simulink model "BANSHEE_SYSTEM"  (Simulink 8.1)
settings: Solver=ode1  StartTime=0.0  StopTime=inf  FixedStep=Ts  MaxStep=1e-3  RelTol=1e-3
PostLoadFcn:
  | Ts=100e-6; BANSHEE_init;
InitFcn:
  | Ts=100e-6; BANSHEE_init;
undefined symbols (not defined in the file or in its folder): cable_spec, F1, F2, F3, Feeder1_lib, Feeder2_lib, Feeder3_lib, Left, relay_housing_lib, SM_UtilityService, SS_F1_RELAY_HOUSING, SS_F2_RELAY_HOUSING, SS_F3_RELAY_HOUSING, SS_Feeder1, SS_Feeder2, SS_Feeder3, type, utility_service_lib, V
libraries: breaker_lib x50, relay_modbus_lib x42, rtio_generic_modbus x42, cables_lib x32, artemis x24, transformer_lib x24, Load_lib x18, ssn_lib x16, rtlab x11, powerlib_extras x3, powerlib x2, LoadProfiles_lib x1
(part 3 of 3)

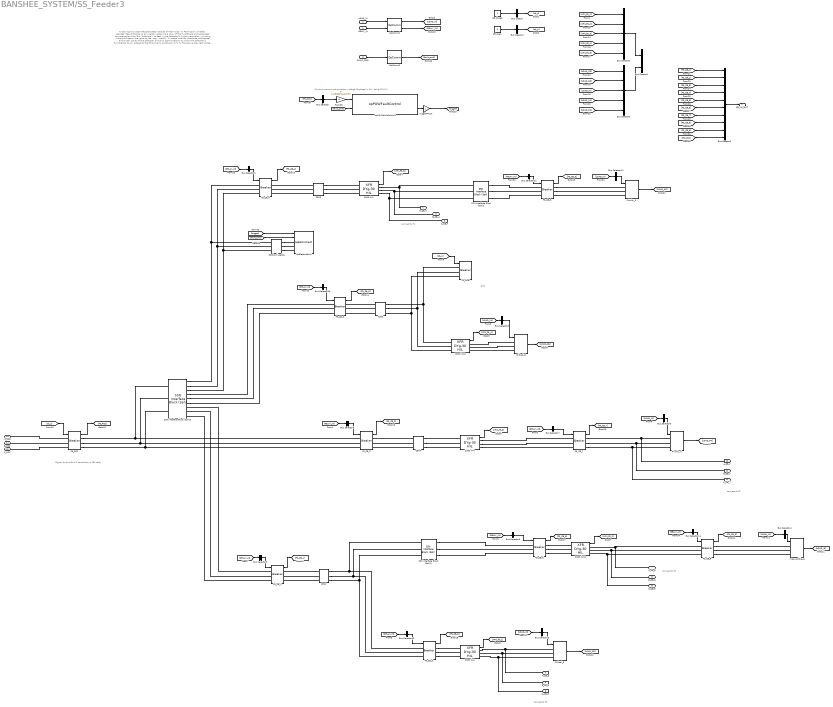
== system BANSHEE_SYSTEM/SS_Feeder3 ==
  note: Signal for this Cb will come from a SEL relay
  note: CHP
  note: connect to F2
  note: connect to F2
  note: connect to F2
  note: connect to F1
  note: % Copyright (c) 2016 Massachusetts Institute of Technology
      | % Permission is hereby granted, free of charge, to any person obtaining a copy of this
      | % software and associated documentation files (the "Software"), to deal in the Software
      | % without restriction, including without limitation the rights to use, copy, modify,
      | % merge, publish, distribute, sublicense, and/or sell copies of the Software, and to
      | % permit persons to whom the Software is furnished to do so, subject to the following
      | % conditions:
      | %
      | %
      | % The above copyright notice and this permission notice shall be included in
      | % all copies or substantial portions of the Software.
      | %
      | % THE SOFTWARE IS PROVIDED "AS IS", WITHOUT WARRANTY OF ANY KIND, EXPRESS OR IMPLIED,
      | % INCLUDING BUT NOT LIMITED TO THE WARRANTIES OF MERCHANTABILITY, FITNESS FOR A
      | % PARTICULAR PURPOSE AND NONINFRINGEMENT. IN NO EVENT SHALL THE AUTHORS OR COPYRIGHT
      | % HOLDERS BE LIABLE FOR ANY CLAIM, DAMAGES OR OTHER LIABILITY, WHETHER IN AN ACTION
      | % OF CONTRACT, TORT OR OTHERWISE, ARISING FROM, OUT OF OR IN CONNECTION WITH THE
      | % SOFTWARE OR THE USE OR OTHER DEALINGS IN THE SOFTWARE.
      | %
      | %
      | %%
  note: Point-on-wave synchronisation voltage (3-phase) in PU - Using 13.8 kV
  RELAY_IN : Inport
  LOAD_IN : Inport  Port=2
  FAULT_CMD : Inport  Port=3
  1000 kVA : transformer_lib/XFR DYg-30 HIL  Rating=1000  Vp=13800  Vs=480  Z=5.56  XR=5.49
  1000 kVA1 : transformer_lib/XFR DYg-30 HIL  Rating=1000  Vp=13800  Vs=480  Z=5.56  XR=5.49
  2000 kVA : transformer_lib/XFR DYg-30 HIL  Rating=2000  Vp=13800  Vs=480  Z=5.75  XR=5.7
  2000 kVA1 : transformer_lib/XFR DYg-30 HIL  Rating=2000  Vp=13800  Vs=480  Z=5.75  XR=5.7
  2500 kVA : transformer_lib/XFR DYg-30 HIL  Rating=2500  Vp=13800  Vs=480  Z=5.75  XR=6.6
  500kcmil_cable : cables_lib/500kcmil_cable  length=1  par_sets=1
  Bus Creator : BusCreator  Inputs=1
  Bus Creator1 : BusCreator  Inputs=1
  Bus Creator2 : BusCreator  Inputs=5
  Bus Creator3 : BusCreator  Inputs=5
  Bus Creator4 : BusCreator  Inputs=2
  Bus Creator5 : BusCreator  Inputs=10
  Bus Selector : BusSelector  OutputSignals=Vabc_bus
  Bus Selector1 : BusSelector  OutputSignals=F3_CB_4
  Bus Selector10 : BusSelector  OutputSignals=F3_CB_5
  Bus Selector11 : BusSelector  OutputSignals=P6
  Bus Selector12 : BusSelector  OutputSignals=F3_CB_9
  Bus Selector13 : BusSelector  OutputSignals=F3_CB_3
  Bus Selector14 : BusSelector  OutputSignals=F3_CB_8
  Bus Selector2 : BusSelector  OutputSignals=C6
  Bus Selector3 : BusSelector  OutputSignals=P4
  Bus Selector4 : BusSelector  OutputSignals=I6
  Bus Selector5 : BusSelector  OutputSignals=C5
  Bus Selector6 : BusSelector  OutputSignals=F3_CB_2
  Bus Selector7 : BusSelector  OutputSignals=F3_CB_7
  Bus Selector8 : BusSelector  OutputSignals=F3_CB_6
  Bus Selector9 : BusSelector  OutputSignals=F3_CB_1
  C301 : cables_lib/PI-Section  cable_spec=[cable_spec(13, :)]  line_length=2500  parallel_sets=1
  C302 : cables_lib/PI-Section  cable_spec=[cable_spec(11, :)]  line_length=2000  parallel_sets=1
  C303 : cables_lib/PI-Section  cable_spec=[cable_spec(13, :)]  line_length=2000  parallel_sets=1
  C304 : cables_lib/PI-Section  cable_spec=[cable_spec(11, :)]  line_length=1500  parallel_sets=2
  CB closed : Constant
  CB open : Constant  Value=0
  Critical_5 : Load_lib/Dynamic_Load  V=460  Ts=Ts
  Critical_6 : Load_lib/Dynamic_Load  V=460  Ts=Ts
  F3_CB_{1..9} (9 alike) : breaker_lib/Breaker  Ts=Ts
  F3_GCB : breaker_lib/Breaker  Ts=Ts
  F3_PCC : breaker_lib/Breaker  Ts=Ts
  Interruptible_6 : Load_lib/Dynamic_Load  V=460  Ts=Ts
  OpComm1 : rtlab/OpComm  nbport=2  groupe_acq=1  subsys_rate=0  st=0  Synchronization=on  Interpolation=on  Threshold=1.0  Missed_Data=off  Sim_Time=off  Samples=off  dynSigOut=off  from_console=0  warning_done=off  writeOpCommFile=off  Offset=off
  OpComm2 : rtlab/OpComm  nbport=1  groupe_acq=1  subsys_rate=0  st=0  Synchronization=on  Interpolation=on  Threshold=1.0  Missed_Data=off  Sim_Time=off  Samples=off  dynSigOut=off  from_console=1  warning_done=off  writeOpCommFile=off  Offset=off
  Priority_4 : Load_lib/Dynamic_Load  V=460  Ts=Ts
  Priority_6 : Load_lib/Dynamic_Load  V=460  Ts=Ts
  SSN Interface Block (3ph)1 : ssn_lib/SSN Interface Block (3ph)  nb_phase=3  nb_port=2  p1_type=V-type(Left)  p2_type=V-type (Right)  p3_type=V-type(Left)  p4_type=V-type(Left)  p5_type=V-type(Left)  p6_type=V-type(Left)  p7_type=V-type(Left)  p8_type=V-type(Left)  p9_type=V-type(Left)  p10_type=V-type(Left)  p11_type=V-type(Left)  p12_type=V-type(Left)  p13_type=V-type(Left)  p14_type=V-type(Left)  p15_type=V-type(Left)  p16_type=V-type(Left)  I_port_shunt_resistance=1e9
  SSN Interface Block (3ph)2 : ssn_lib/SSN Interface Block (3ph)  nb_phase=3  nb_port=2  p1_type=V-type(Left)  p2_type=V-type (Right)  p3_type=V-type(Left)  p4_type=V-type(Left)  p5_type=V-type(Left)  p6_type=V-type(Left)  p7_type=V-type(Left)  p8_type=V-type(Left)  p9_type=V-type(Left)  p10_type=V-type(Left)  p11_type=V-type(Left)  p12_type=V-type(Left)  p13_type=V-type(Left)  p14_type=V-type(Left)  p15_type=V-type(Left)  p16_type=V-type(Left)  I_port_shunt_resistance=1e9
  SSN Interface Block (3ph)5 : ssn_lib/SSN Interface Block (3ph)  nb_phase=3  nb_port=4  p1_type=V-type(Left)  p2_type=V-type (Right)  p3_type=V-type (Right)  p4_type=V-type (Right)  p5_type=V-type(Left)  p6_type=V-type(Left)  p7_type=V-type(Left)  p8_type=V-type(Left)  p9_type=V-type(Left)  p10_type=V-type(Left)  p11_type=V-type(Left)  p12_type=V-type(Left)  p13_type=V-type(Left)  p14_type=V-type(Left)  p15_type=V-type(Left)  p16_type=V-type(Left)  I_port_shunt_resistance=1e9
  a : Gain  Gain=1/(13800*sqrt(2/3))
  opElectricFault : artemis/Tools /POW faults/opElectricFault  FaultLocation=location 4  FaultResistance=0.0001  GroundResistance=0.0001  InitialStates=[0 0 0]  SnubberResistance=1e6  SnubberCapacitance=inf
  opPOWFaultControl1 : artemis/Tools /POW faults/opPOWFaultControl  Ts=Ts  usePLL=off  Fgrid=60  PLL_k=[180 3200 1]  vol_sel=1: rising zero-corssing  SyncPhase_menu=A  T_acq=0.8
  triggerFAULT : Gain
  A_CB_4 : PMIOPort  Port=1  Side=Right
  B_CB_4 : PMIOPort  Port=2  Side=Right
  C_CB_4 : PMIOPort  Port=3  Side=Right
  A_CB_5 : PMIOPort  Port=4  Side=Right
  B_CB_5 : PMIOPort  Port=5  Side=Right
  C_CB_5 : PMIOPort  Port=6  Side=Right
  A_CB_6 : PMIOPort  Port=7  Side=Right
  B_CB_6 : PMIOPort  Port=8  Side=Right
  C_CB_6 : PMIOPort  Port=9  Side=Right
  A_CB_7 : PMIOPort  Port=10  Side=Right
  B_CB_7 : PMIOPort  Port=11  Side=Right
  C_CB_7 : PMIOPort  Port=12  Side=Right
  A_PCC : PMIOPort  Port=13  Side=Left
  B_PCC : PMIOPort  Port=14  Side=Left
  C_PCC : PMIOPort  Port=15  Side=Left
  CB_MS_OUT : Outport
  wires:
  CB closed/1 -> Bus Creator/1  "Logic_trip"
  Bus Creator/1 -> [cb_c]
  Bus Creator1/1 -> [cb_o]
  Bus Selector1/1 -> F3_CB_4/1  "<F3_CB_4>"
  CB open/1 -> Bus Creator1/1  "Logic_trip"
  LOAD_IN/1 -> OpComm1/1
  OpComm1/1 -> [LOAD_IN]
  [LOAD_IN] -> Bus Selector2/1
  [LOAD_IN] -> Bus Selector3/1
  [LOAD_IN] -> Bus Selector4/1
  [LOAD_IN] -> Bus Selector5/1
  Bus Selector2/1 -> Critical_6/1  "<C6>"
  Bus Selector3/1 -> Priority_4/1  "<P4>"
  Bus Selector4/1 -> Interruptible_6/1  "<I6>"
  Bus Selector5/1 -> Critical_5/1  "<C5>"
  2000 kVA/1 -> [XFM_F3_1]
  2000 kVA1/1 -> [XFM_F3_2]
  1000 kVA/1 -> [XFM_F3_3]
  1000 kVA1/1 -> [XFM_F3_4]
  [XFM_F3_2] -> Bus Creator2/2  "F3_X2"
  [XFM_F3_1] -> Bus Creator2/1  "F3_X1"
  [XFM_F3_5] -> Bus Creator2/5  "F3_X5"
  [XFM_F3_3] -> Bus Creator2/3  "F3_X3"
  [XFM_F3_4] -> Bus Creator2/4  "F3_X4"
  Critical_6/1 -> [LOAD_C6]
  Priority_4/1 -> [LOAD_P4]
  Interruptible_6/1 -> [LOAD_I6]
  Critical_5/1 -> [LOAD_C5]
  [LOAD_C6] -> Bus Creator3/2  "F3_C6"
  [LOAD_C5] -> Bus Creator3/1  "F3_C5"
  [LOAD_I6] -> Bus Creator3/3  "F3_I6"
  [LOAD_P4] -> Bus Creator3/4  "F3_P4"
  Bus Creator2/1 -> Bus Creator4/1  "XFR"
  Bus Creator3/1 -> Bus Creator4/2  "LOAD"
  F3_CB_4/1 -> [F3_CB_4]
  F3_CB_3/1 -> [F3_CB_3]
  F3_CB_2/1 -> [F3_CB_2]
  F3_CB_6/1 -> [F3_CB_6]
  F3_CB_1/1 -> [F3_CB_1]
  F3_CB_5/1 -> [F3_CB_5]
  [F3_CB_1] -> Bus Creator5/1  "F3_CB_1"
  [F3_CB_5] -> Bus Creator5/5  "F3_CB_5"
  [F3_CB_7] -> Bus Creator5/7  "F3_CB_7"
  [F3_CB_6] -> Bus Creator5/6  "F3_CB_6"
  [F3_CB_3] -> Bus Creator5/3  "F3_CB_3"
  [F3_CB_2] -> Bus Creator5/2  "F3_CB_2"
  [F3_CB_4] -> Bus Creator5/4  "F3_CB_4"
  Bus Creator5/1 -> CB_MS_OUT/1
  [RELAY_IN] -> Bus Selector1/1
  RELAY_IN/1 -> OpComm1/2
  OpComm1/2 -> [RELAY_IN]
  Bus Selector6/1 -> F3_CB_2/1  "<F3_CB_2>"
  [RELAY_IN] -> Bus Selector6/1
  Bus Selector7/1 -> F3_CB_7/1  "<F3_CB_7>"
  [RELAY_IN] -> Bus Selector7/1
  Bus Selector8/1 -> F3_CB_6/1  "<F3_CB_6>"
  [RELAY_IN] -> Bus Selector8/1
  Bus Selector9/1 -> F3_CB_1/1  "<F3_CB_1>"
  [RELAY_IN] -> Bus Selector9/1
  Bus Selector10/1 -> F3_CB_5/1  "<F3_CB_5>"
  [RELAY_IN] -> Bus Selector10/1
  Bus Selector13/1 -> F3_CB_3/1  "<F3_CB_3>"
  [RELAY_IN] -> Bus Selector13/1
  [cb_c] -> F3_PCC/1
  [cb_o] -> F3_GCB/1
  2500 kVA/1 -> [XFM_F3_5]
  F3_CB_7/1 -> [F3_CB_7]
  F3_PCC/1 -> [F3_PCC]
  [F3_PCC] -> Bus Creator5/10  "F3_PCC"
  [LOAD_IN] -> Bus Selector11/1
  Bus Selector11/1 -> Priority_6/1  "<P6>"
  Priority_6/1 -> [LOAD_P6]
  [LOAD_P6] -> Bus Creator3/5  "F3_P6"
  F3_CB_9/1 -> [F3_CB_9]
  Bus Selector12/1 -> F3_CB_9/1  "<F3_CB_9>"
  [RELAY_IN] -> Bus Selector12/1
  F3_CB_8/1 -> [F3_CB_8]
  Bus Selector14/1 -> F3_CB_8/1  "<F3_CB_8>"
  [RELAY_IN] -> Bus Selector14/1
  [F3_CB_8] -> Bus Creator5/8  "F3_CB_8"
  [F3_CB_9] -> Bus Creator5/9  "F3_CB_9"
  [fault_cmd] -> opPOWFaultControl1/2
  opPOWFaultControl1/2 -> triggerFAULT/1
  triggerFAULT/1 -> [trigger]  "triggerFAULTsig"
  [F3_PCC] -> Bus Selector/1
  Bus Selector/1 -> a/1  "<Vabc_bus>"
  a/1 -> opPOWFaultControl1/1
  [fault_cmd] -> opElectricFault/2
  [trigger] -> opElectricFault/1
  OpComm2/1 -> [fault_cmd]
  FAULT_CMD/1 -> OpComm2/1
  connections:
  F3_CB_5/LConn1 -- C301/RConn1 -- SSN Interface Block (3ph)1/LConn1
  F3_CB_6/RConn3 -- 2000 kVA1/LConn3
  Critical_6/LConn2 -- 1000 kVA1/RConn2
  C301/LConn2 -- F3_CB_1/RConn2
  Critical_6/LConn1 -- 1000 kVA1/RConn1
  F3_CB_5/LConn3 -- C301/RConn3 -- SSN Interface Block (3ph)1/LConn3
  Critical_6/LConn3 -- 1000 kVA1/RConn3
  C301/LConn3 -- F3_CB_1/RConn3
  C304/LConn1 -- F3_CB_2/RConn1
  1000 kVA1/LConn3 -- C302/RConn3 -- F3_GCB/LConn3
  C302/LConn2 -- F3_CB_3/RConn2
  1000 kVA1/LConn1 -- C302/RConn1 -- F3_GCB/LConn1
  F3_CB_6/RConn2 -- 2000 kVA1/LConn2
  1000 kVA1/LConn2 -- C302/RConn2 -- F3_GCB/LConn2
  C301/LConn1 -- F3_CB_1/RConn1
  F3_CB_5/RConn2 -- 2000 kVA/LConn2
  C302/LConn3 -- F3_CB_3/RConn3
  F3_CB_5/LConn2 -- C301/RConn2 -- SSN Interface Block (3ph)1/LConn2
  C304/LConn2 -- F3_CB_2/RConn2
  F3_CB_6/RConn1 -- 2000 kVA1/LConn1
  C302/LConn1 -- F3_CB_3/RConn1
  F3_CB_5/RConn1 -- 2000 kVA/LConn1
  F3_CB_5/RConn3 -- 2000 kVA/LConn3
  C304/LConn3 -- F3_CB_2/RConn3
  F3_CB_7/RConn1 -- A_CB_7/RConn1 -- Priority_4/LConn1
  F3_CB_7/RConn3 -- C_CB_7/RConn1 -- Priority_4/LConn3
  F3_CB_7/RConn2 -- B_CB_7/RConn1 -- Priority_4/LConn2
  F3_CB_8/LConn1 -- A_CB_6/RConn1 -- 2000 kVA1/RConn1
  2000 kVA1/RConn3 -- C_CB_6/RConn1 -- F3_CB_8/LConn3
  F3_CB_8/LConn2 -- B_CB_6/RConn1 -- 2000 kVA1/RConn2
  Critical_5/LConn1 -- A_CB_5/RConn1 -- 2000 kVA/RConn1
  2000 kVA/RConn3 -- C_CB_5/RConn1 -- Critical_5/LConn3
  2000 kVA/RConn2 -- B_CB_5/RConn1 -- Critical_5/LConn2
  2500 kVA/RConn1 -- SSN Interface Block (3ph)2/LConn1 -- A_CB_4/RConn1
  2500 kVA/RConn3 -- SSN Interface Block (3ph)2/LConn3 -- C_CB_4/RConn1
  2500 kVA/RConn2 -- SSN Interface Block (3ph)2/LConn2 -- B_CB_4/RConn1
  C304/RConn2 -- 1000 kVA/LConn2
  C304/RConn3 -- 1000 kVA/LConn3
  C304/RConn1 -- 1000 kVA/LConn1
  1000 kVA/RConn3 -- F3_CB_7/LConn3
  1000 kVA/RConn2 -- F3_CB_7/LConn2
  1000 kVA/RConn1 -- F3_CB_7/LConn1
  F3_CB_9/RConn1 -- Priority_6/LConn1
  F3_CB_9/RConn2 -- Priority_6/LConn2
  F3_CB_9/RConn3 -- Priority_6/LConn3
  F3_CB_8/RConn1 -- Interruptible_6/LConn1
  F3_CB_8/RConn2 -- Interruptible_6/LConn2
  F3_CB_8/RConn3 -- Interruptible_6/LConn3
  SSN Interface Block (3ph)5/RConn1 -- 500kcmil_cable/LConn1 -- F3_CB_4/LConn1
  SSN Interface Block (3ph)5/RConn3 -- 500kcmil_cable/LConn3 -- F3_CB_4/LConn3
  SSN Interface Block (3ph)5/RConn2 -- 500kcmil_cable/LConn2 -- F3_CB_4/LConn2
  SSN Interface Block (3ph)5/RConn4 -- F3_CB_3/LConn1
  SSN Interface Block (3ph)5/RConn6 -- F3_CB_3/LConn3
  SSN Interface Block (3ph)5/RConn5 -- F3_CB_3/LConn2
  F3_CB_1/LConn1 -- SSN Interface Block (3ph)5/RConn7
  F3_CB_1/LConn2 -- SSN Interface Block (3ph)5/RConn8
  F3_CB_1/LConn3 -- SSN Interface Block (3ph)5/RConn9
  SSN Interface Block (3ph)1/RConn2 -- F3_CB_6/LConn2
  SSN Interface Block (3ph)1/RConn1 -- F3_CB_6/LConn1
  SSN Interface Block (3ph)1/RConn3 -- F3_CB_6/LConn3
  C303/LConn1 -- F3_CB_4/RConn1
  C303/LConn2 -- F3_CB_4/RConn2
  C303/LConn3 -- F3_CB_4/RConn3
  C303/RConn2 -- 2500 kVA/LConn2
  C303/RConn3 -- 2500 kVA/LConn3
  C303/RConn1 -- 2500 kVA/LConn1
  F3_PCC/LConn2 -- B_PCC/RConn1
  F3_PCC/LConn3 -- C_PCC/RConn1
  F3_PCC/LConn1 -- A_PCC/RConn1
  F3_PCC/RConn1 -- F3_CB_2/LConn1 -- SSN Interface Block (3ph)5/LConn1
  F3_PCC/RConn3 -- F3_CB_2/LConn3 -- SSN Interface Block (3ph)5/LConn3
  F3_PCC/RConn2 -- F3_CB_2/LConn2 -- SSN Interface Block (3ph)5/LConn2
  500kcmil_cable/RConn2 -- opElectricFault/LConn2
  500kcmil_cable/RConn3 -- opElectricFault/LConn3
  500kcmil_cable/RConn1 -- opElectricFault/LConn1
  SSN Interface Block (3ph)2/RConn2 -- F3_CB_9/LConn2
  SSN Interface Block (3ph)2/RConn3 -- F3_CB_9/LConn3
  SSN Interface Block (3ph)2/RConn1 -- F3_CB_9/LConn1

== system BANSHEE_SYSTEM/SC_ctrl/Overall ==
  F1 : Inport
  F2 : Inport  Port=2
  F3 : Inport  Port=3
  Iabc : Scope  NumInputPorts=3
      settings: ShowLegends=on  TimeRange=10  YMin=0~0~2  YMax=47.5~650~21  Decimation=10
  Vpu : Scope  NumInputPorts=3
      settings: ShowLegends=on  TimeRange=10  YMin=0~0~0  YMax=1.4~1.4~1.4  SaveName=ScopeData3  Decimation=10
  currents : Subsystem
  voltages : Subsystem
  wires:
  voltages/1(oF1) -> Vpu/1
  voltages/2(oF2) -> Vpu/2
  voltages/3(oF3) -> Vpu/3
  currents/1(oF1) -> Iabc/1
  currents/2(oF2) -> Iabc/2
  currents/3(oF3) -> Iabc/3
  F3/1 -> voltages/3(F3), currents/3(F3)
  F2/1 -> currents/2(F2), voltages/2(F2)
  F1/1 -> voltages/1(F1), currents/1(F1)

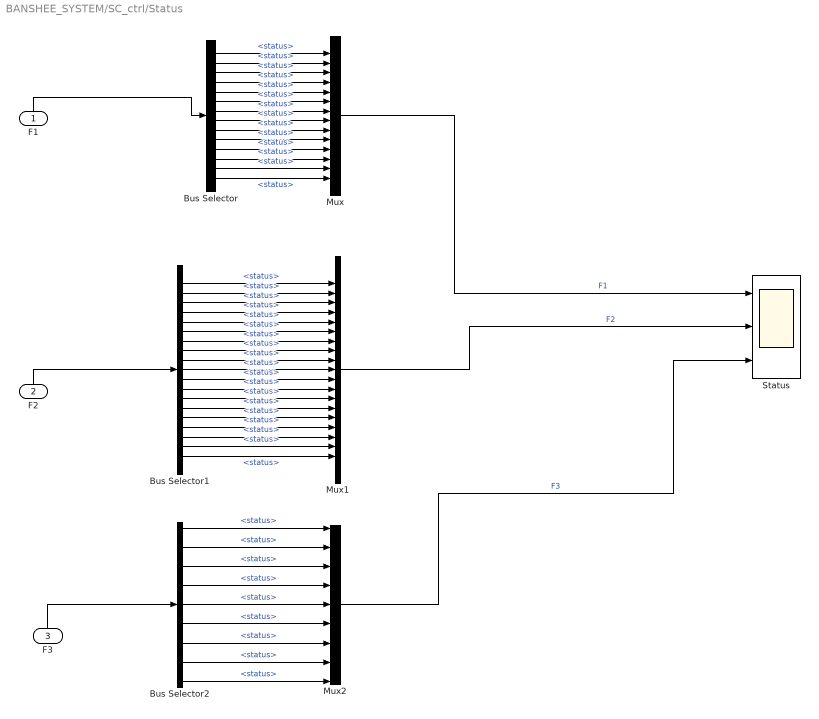
== system BANSHEE_SYSTEM/SC_ctrl/Status ==
  F1 : Inport
  F2 : Inport  Port=2
  F3 : Inport  Port=3
  Bus Selector : BusSelector  OutputSignals=F1_CB_1.m.status,F1_CB_2.m.status,F1_CB_3.m.status,F1_CB_4.m.status,F1_CB_5.m.status,F1_CB_6.m.status,F1_CB_7.m.status,F1_CB_8.m.status,F1_CB_9.m.status,F1_CB_10.m.status,F1_CB_11.m.status,F1_CB_12.m.status,F1_CB_13.m.status,F1_CB_14.m.status
  Bus Selector1 : BusSelector  OutputSignals=F2_CB_1.m.status,F2_CB_2.m.status,F2_CB_3.m.status,F2_CB_4.m.status,F2_CB_5.m.status,F2_CB_6.m.status,F2_CB_7.m.status,F2_CB_8.m.status,F2_CB_9.m.status,F2_CB_10.m.status,F2_CB_11.m.status,F2_CB_12.m.status,F2_CB_13.m.status,F2_CB_14.m.status,F2_CB_15.m.status,F2_CB_16.m.status,F2_CB_17.m.status,F2_CB_18.m.status,F2_CB_19.m.status
  Bus Selector2 : BusSelector  OutputSignals=F3_CB_1.m.status,F3_CB_2.m.status,F3_CB_3.m.status,F3_CB_4.m.status,F3_CB_5.m.status,F3_CB_6.m.status,F3_CB_7.m.status,F3_CB_8.m.status,F3_CB_9.m.status
  Mux : Mux  Inputs=14
  Mux1 : Mux  Inputs=19
  Mux2 : Mux  Inputs=9
  Status : Scope  NumInputPorts=3
      settings: ShowLegends=on  TimeRange=0.4  YMin=2~2~2.85  YMax=3~19~3.15  SaveName=ScopeData3  Decimation=20
  wires:
  Mux/1 -> Status/1  "F1"
  F1/1 -> Bus Selector/1
  Mux1/1 -> Status/2  "F2"
  F2/1 -> Bus Selector1/1
  Mux2/1 -> Status/3  "F3"
  F3/1 -> Bus Selector2/1
  Bus Selector1/3 -> Mux1/3  "<status>"
  Bus Selector1/13 -> Mux1/13  "<status>"
  Bus Selector1/8 -> Mux1/8  "<status>"
  Bus Selector1/4 -> Mux1/4  "<status>"
  Bus Selector1/6 -> Mux1/6  "<status>"
  Bus Selector1/2 -> Mux1/2  "<status>"
  Bus Selector1/7 -> Mux1/7  "<status>"
  Bus Selector1/10 -> Mux1/10  "<status>"
  Bus Selector1/12 -> Mux1/12  "<status>"
  Bus Selector1/1 -> Mux1/1  "<status>"
  Bus Selector1/5 -> Mux1/5  "<status>"
  Bus Selector1/14 -> Mux1/14  "<status>"
  Bus Selector1/9 -> Mux1/9  "<status>"
  Bus Selector1/11 -> Mux1/11  "<status>"
  Bus Selector1/17 -> Mux1/17  "<status>"
  Bus Selector1/16 -> Mux1/16  "<status>"
  Bus Selector1/15 -> Mux1/15  "<status>"
  Bus Selector1/18 -> Mux1/18  "<status>"
  Bus Selector1/19 -> Mux1/19  "<status>"
  Bus Selector/4 -> Mux/4  "<status>"
  Bus Selector/10 -> Mux/10  "<status>"
  Bus Selector/8 -> Mux/8  "<status>"
  Bus Selector/1 -> Mux/1  "<status>"
  Bus Selector/7 -> Mux/7  "<status>"
  Bus Selector/12 -> Mux/12  "<status>"
  Bus Selector/5 -> Mux/5  "<status>"
  Bus Selector/9 -> Mux/9  "<status>"
  Bus Selector/2 -> Mux/2  "<status>"
  Bus Selector/3 -> Mux/3  "<status>"
  Bus Selector/6 -> Mux/6  "<status>"
  Bus Selector/11 -> Mux/11  "<status>"
  Bus Selector/13 -> Mux/13  "<status>"
  Bus Selector/14 -> Mux/14  "<status>"
  Bus Selector2/6 -> Mux2/6  "<status>"
  Bus Selector2/5 -> Mux2/5  "<status>"
  Bus Selector2/7 -> Mux2/7  "<status>"
  Bus Selector2/4 -> Mux2/4  "<status>"
  Bus Selector2/8 -> Mux2/8  "<status>"
  Bus Selector2/3 -> Mux2/3  "<status>"
  Bus Selector2/9 -> Mux2/9  "<status>"
  Bus Selector2/2 -> Mux2/2  "<status>"
  Bus Selector2/1 -> Mux2/1  "<status>"

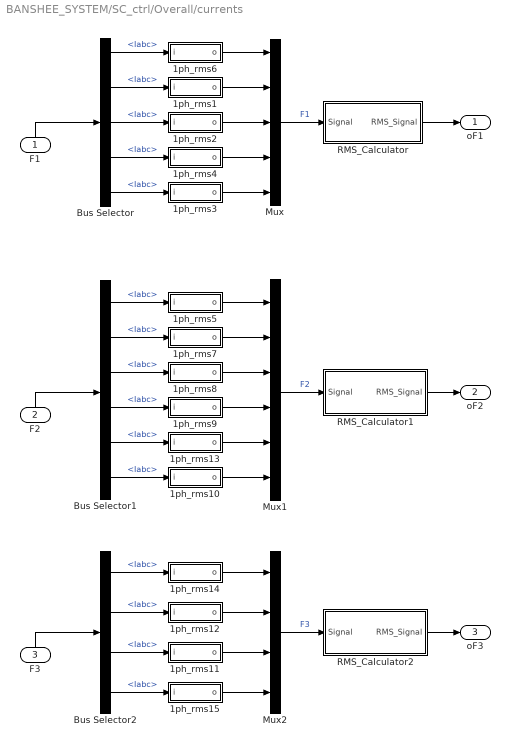
== system BANSHEE_SYSTEM/SC_ctrl/Overall/currents ==
  F1 : Inport
  F2 : Inport  Port=2
  F3 : Inport  Port=3
  1ph_rms1 : Subsystem
  1ph_rms10 : Subsystem
  1ph_rms11 : Subsystem
  1ph_rms12 : Subsystem
  1ph_rms13 : Subsystem
  1ph_rms14 : Subsystem
  1ph_rms15 : Subsystem
  1ph_rms2 : Subsystem
  1ph_rms3 : Subsystem
  1ph_rms4 : Subsystem
  1ph_rms5 : Subsystem
  1ph_rms6 : Subsystem
  1ph_rms7 : Subsystem
  1ph_rms8 : Subsystem
  1ph_rms9 : Subsystem
  Bus Selector : BusSelector  OutputSignals=F1_CB_1.m.Iabc,F1_CB_2.m.Iabc,F1_CB_3.m.Iabc,F1_CB_6.m.Iabc,F1_CB_10.m.Iabc
  Bus Selector1 : BusSelector  OutputSignals=F2_CB_1.m.Iabc,F2_CB_2.m.Iabc,F2_CB_3.m.Iabc,F2_CB_7.m.Iabc,F2_CB_14.m.Iabc,F2_CB_15.m.Iabc
  Bus Selector2 : BusSelector  OutputSignals=F3_CB_1.m.Iabc,F3_CB_2.m.Iabc,F3_CB_3.m.Iabc,F3_CB_4.m.Iabc
  Mux : Mux  Inputs=5
  Mux1 : Mux  Inputs=6
  Mux2 : Mux
  RMS_Calculator : Subsystem
  RMS_Calculator1 : Subsystem
  RMS_Calculator2 : Subsystem
  oF1 : Outport
  oF2 : Outport  Port=2
  oF3 : Outport  Port=3
  wires:
  Mux/1 -> RMS_Calculator/1(Signal)  "F1"
  Mux1/1 -> RMS_Calculator1/1(Signal)  "F2"
  Mux2/1 -> RMS_Calculator2/1(Signal)  "F3"
  Bus Selector/5 -> 1ph_rms3/1(i)  "<Iabc>"
  Bus Selector/4 -> 1ph_rms4/1(i)  "<Iabc>"
  Bus Selector/3 -> 1ph_rms2/1(i)  "<Iabc>"
  Bus Selector/2 -> 1ph_rms1/1(i)  "<Iabc>"
  Bus Selector/1 -> 1ph_rms6/1(i)  "<Iabc>"
  Bus Selector1/4 -> 1ph_rms9/1(i)  "<Iabc>"
  Bus Selector1/5 -> 1ph_rms13/1(i)  "<Iabc>"
  Bus Selector1/3 -> 1ph_rms8/1(i)  "<Iabc>"
  Bus Selector1/6 -> 1ph_rms10/1(i)  "<Iabc>"
  Bus Selector1/2 -> 1ph_rms7/1(i)  "<Iabc>"
  Bus Selector1/1 -> 1ph_rms5/1(i)  "<Iabc>"
  Bus Selector2/4 -> 1ph_rms15/1(i)  "<Iabc>"
  Bus Selector2/2 -> 1ph_rms12/1(i)  "<Iabc>"
  Bus Selector2/3 -> 1ph_rms11/1(i)  "<Iabc>"
  Bus Selector2/1 -> 1ph_rms14/1(i)  "<Iabc>"
  1ph_rms6/1(o) -> Mux/1
  1ph_rms1/1(o) -> Mux/2
  1ph_rms2/1(o) -> Mux/3
  1ph_rms3/1(o) -> Mux/5
  1ph_rms4/1(o) -> Mux/4
  1ph_rms5/1(o) -> Mux1/1
  1ph_rms7/1(o) -> Mux1/2
  1ph_rms8/1(o) -> Mux1/3
  1ph_rms9/1(o) -> Mux1/4
  1ph_rms14/1(o) -> Mux2/1
  1ph_rms13/1(o) -> Mux1/5
  1ph_rms10/1(o) -> Mux1/6
  1ph_rms12/1(o) -> Mux2/2
  1ph_rms11/1(o) -> Mux2/3
  1ph_rms15/1(o) -> Mux2/4
  RMS_Calculator/1(RMS_Signal) -> oF1/1
  RMS_Calculator1/1(RMS_Signal) -> oF2/1
  RMS_Calculator2/1(RMS_Signal) -> oF3/1
  F1/1 -> Bus Selector/1
  F2/1 -> Bus Selector1/1
  F3/1 -> Bus Selector2/1

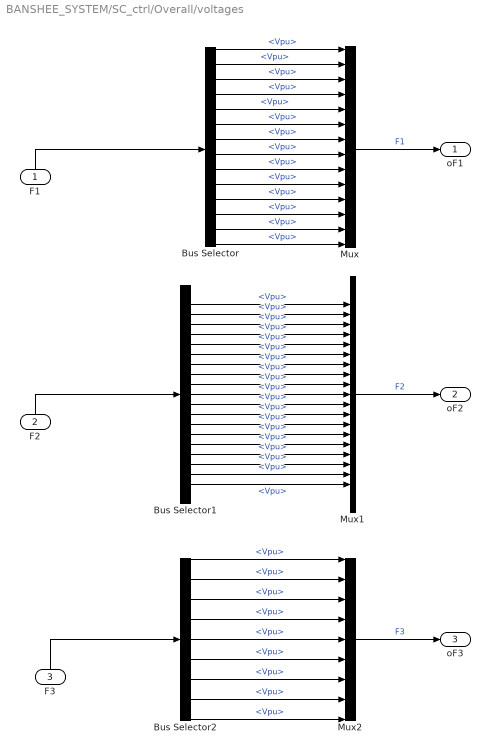
== system BANSHEE_SYSTEM/SC_ctrl/Overall/voltages ==
  F1 : Inport
  F2 : Inport  Port=2
  F3 : Inport  Port=3
  Bus Selector : BusSelector  OutputSignals=F1_CB_1.m.Vpu,F1_CB_2.m.Vpu,F1_CB_3.m.Vpu,F1_CB_4.m.Vpu,F1_CB_5.m.Vpu,F1_CB_6.m.Vpu,F1_CB_7.m.Vpu,F1_CB_8.m.Vpu,F1_CB_9.m.Vpu,F1_CB_10.m.Vpu,F1_CB_11.m.Vpu,F1_CB_12.m.Vpu,F1_CB_13.m.Vpu,F1_CB_14.m.Vpu
  Bus Selector1 : BusSelector  OutputSignals=F2_CB_1.m.Vpu,F2_CB_2.m.Vpu,F2_CB_3.m.Vpu,F2_CB_4.m.Vpu,F2_CB_5.m.Vpu,F2_CB_6.m.Vpu,F2_CB_7.m.Vpu,F2_CB_8.m.Vpu,F2_CB_9.m.Vpu,F2_CB_10.m.Vpu,F2_CB_11.m.Vpu,F2_CB_12.m.Vpu,F2_CB_13.m.Vpu,F2_CB_14.m.Vpu,F2_CB_15.m.Vpu,F2_CB_16.m.Vpu,F2_CB_17.m.Vpu,F2_CB_18.m.Vpu,F2_CB_19.m.Vpu
  Bus Selector2 : BusSelector  OutputSignals=F3_CB_1.m.Vpu,F3_CB_2.m.Vpu,F3_CB_3.m.Vpu,F3_CB_4.m.Vpu,F3_CB_5.m.Vpu,F3_CB_6.m.Vpu,F3_CB_7.m.Vpu,F3_CB_8.m.Vpu,F3_CB_9.m.Vpu
  Mux : Mux  Inputs=14
  Mux1 : Mux  Inputs=19
  Mux2 : Mux  Inputs=9
  oF1 : Outport
  oF2 : Outport  Port=2
  oF3 : Outport  Port=3
  wires:
  Mux/1 -> oF1/1  "F1"
  F1/1 -> Bus Selector/1
  Mux1/1 -> oF2/1  "F2"
  F2/1 -> Bus Selector1/1
  Mux2/1 -> oF3/1  "F3"
  F3/1 -> Bus Selector2/1
  Bus Selector/14 -> Mux/14  "<Vpu>"
  Bus Selector/6 -> Mux/6  "<Vpu>"
  Bus Selector/5 -> Mux/5  "<Vpu>"
  Bus Selector/10 -> Mux/10  "<Vpu>"
  Bus Selector/4 -> Mux/4  "<Vpu>"
  Bus Selector/9 -> Mux/9  "<Vpu>"
  Bus Selector/7 -> Mux/7  "<Vpu>"
  Bus Selector/2 -> Mux/2  "<Vpu>"
  Bus Selector/1 -> Mux/1  "<Vpu>"
  Bus Selector/3 -> Mux/3  "<Vpu>"
  Bus Selector/13 -> Mux/13  "<Vpu>"
  Bus Selector/12 -> Mux/12  "<Vpu>"
  Bus Selector/11 -> Mux/11  "<Vpu>"
  Bus Selector/8 -> Mux/8  "<Vpu>"
  Bus Selector1/19 -> Mux1/19  "<Vpu>"
  Bus Selector1/18 -> Mux1/18  "<Vpu>"
  Bus Selector1/7 -> Mux1/7  "<Vpu>"
  Bus Selector1/10 -> Mux1/10  "<Vpu>"
  Bus Selector1/11 -> Mux1/11  "<Vpu>"
  Bus Selector1/2 -> Mux1/2  "<Vpu>"
  Bus Selector1/13 -> Mux1/13  "<Vpu>"
  Bus Selector1/14 -> Mux1/14  "<Vpu>"
  Bus Selector1/15 -> Mux1/15  "<Vpu>"
  Bus Selector1/6 -> Mux1/6  "<Vpu>"
  Bus Selector1/4 -> Mux1/4  "<Vpu>"
  Bus Selector1/3 -> Mux1/3  "<Vpu>"
  Bus Selector1/1 -> Mux1/1  "<Vpu>"
  Bus Selector1/5 -> Mux1/5  "<Vpu>"
  Bus Selector1/8 -> Mux1/8  "<Vpu>"
  Bus Selector1/12 -> Mux1/12  "<Vpu>"
  Bus Selector1/16 -> Mux1/16  "<Vpu>"
  Bus Selector1/17 -> Mux1/17  "<Vpu>"
  Bus Selector1/9 -> Mux1/9  "<Vpu>"
  Bus Selector2/5 -> Mux2/5  "<Vpu>"
  Bus Selector2/4 -> Mux2/4  "<Vpu>"
  Bus Selector2/6 -> Mux2/6  "<Vpu>"
  Bus Selector2/3 -> Mux2/3  "<Vpu>"
  Bus Selector2/7 -> Mux2/7  "<Vpu>"
  Bus Selector2/8 -> Mux2/8  "<Vpu>"
  Bus Selector2/2 -> Mux2/2  "<Vpu>"
  Bus Selector2/9 -> Mux2/9  "<Vpu>"
  Bus Selector2/1 -> Mux2/1  "<Vpu>"

== system BANSHEE_SYSTEM/SC_ctrl/Overall/currents/1ph_rms1 ==
  i : Inport
  Demux : Demux  Outputs=3
  o : Outport
  wires:
  Demux/1 -> o/1
  i/1 -> Demux/1

== system BANSHEE_SYSTEM/SC_ctrl/Overall/currents/1ph_rms10 ==
  i : Inport
  Demux : Demux  Outputs=3
  o : Outport
  wires:
  Demux/1 -> o/1
  i/1 -> Demux/1

== system BANSHEE_SYSTEM/SC_ctrl/Overall/currents/1ph_rms11 ==
  i : Inport
  Demux : Demux  Outputs=3
  o : Outport
  wires:
  Demux/1 -> o/1
  i/1 -> Demux/1

== system BANSHEE_SYSTEM/SC_ctrl/Overall/currents/1ph_rms12 ==
  i : Inport
  Demux : Demux  Outputs=3
  o : Outport
  wires:
  Demux/1 -> o/1
  i/1 -> Demux/1

== system BANSHEE_SYSTEM/SC_ctrl/Overall/currents/1ph_rms13 ==
  i : Inport
  Demux : Demux  Outputs=3
  o : Outport
  wires:
  Demux/1 -> o/1
  i/1 -> Demux/1

== system BANSHEE_SYSTEM/SC_ctrl/Overall/currents/1ph_rms14 ==
  i : Inport
  Demux : Demux  Outputs=3
  o : Outport
  wires:
  Demux/1 -> o/1
  i/1 -> Demux/1

== system BANSHEE_SYSTEM/SC_ctrl/Overall/currents/1ph_rms15 ==
  i : Inport
  Demux : Demux  Outputs=3
  o : Outport
  wires:
  Demux/1 -> o/1
  i/1 -> Demux/1

== system BANSHEE_SYSTEM/SC_ctrl/Overall/currents/1ph_rms2 ==
  i : Inport
  Demux : Demux  Outputs=3
  o : Outport
  wires:
  Demux/1 -> o/1
  i/1 -> Demux/1

== system BANSHEE_SYSTEM/SC_ctrl/Overall/currents/1ph_rms3 ==
  i : Inport
  Demux : Demux  Outputs=3
  o : Outport
  wires:
  Demux/1 -> o/1
  i/1 -> Demux/1

== system BANSHEE_SYSTEM/SC_ctrl/Overall/currents/1ph_rms4 ==
  i : Inport
  Demux : Demux  Outputs=3
  o : Outport
  wires:
  Demux/1 -> o/1
  i/1 -> Demux/1

== system BANSHEE_SYSTEM/SC_ctrl/Overall/currents/1ph_rms5 ==
  i : Inport
  Demux : Demux  Outputs=3
  o : Outport
  wires:
  Demux/1 -> o/1
  i/1 -> Demux/1

== system BANSHEE_SYSTEM/SC_ctrl/Overall/currents/1ph_rms6 ==
  i : Inport
  Demux : Demux  Outputs=3
  o : Outport
  wires:
  Demux/1 -> o/1
  i/1 -> Demux/1

== system BANSHEE_SYSTEM/SC_ctrl/Overall/currents/1ph_rms7 ==
  i : Inport
  Demux : Demux  Outputs=3
  o : Outport
  wires:
  Demux/1 -> o/1
  i/1 -> Demux/1

== system BANSHEE_SYSTEM/SC_ctrl/Overall/currents/1ph_rms8 ==
  i : Inport
  Demux : Demux  Outputs=3
  o : Outport
  wires:
  Demux/1 -> o/1
  i/1 -> Demux/1

== system BANSHEE_SYSTEM/SC_ctrl/Overall/currents/1ph_rms9 ==
  i : Inport
  Demux : Demux  Outputs=3
  o : Outport
  wires:
  Demux/1 -> o/1
  i/1 -> Demux/1

== system BANSHEE_SYSTEM/SC_ctrl/Overall/currents/RMS_Calculator ==
  Signal : Inport
  Discrete  Mean value6 : powerlib_extras/Discrete Measurements/Discrete  Mean value  Freq=60  Vinit=0  Ts=Ts
  Product3 : Product  RndMeth=Zero
  Signed Sqrt : Sqrt  SaturateOnIntegerOverflow=on
  RMS_Signal : Outport
  wires:
  Signed Sqrt/1 -> RMS_Signal/1
  Discrete  Mean value6/1 -> Signed Sqrt/1
  Product3/1 -> Discrete  Mean value6/1
  Signal/1 -> Product3/2, Product3/1

== system BANSHEE_SYSTEM/SC_ctrl/Overall/currents/RMS_Calculator1 ==
  Signal : Inport
  Discrete  Mean value6 : powerlib_extras/Discrete Measurements/Discrete  Mean value  Freq=60  Vinit=0  Ts=Ts
  Product3 : Product  RndMeth=Zero
  Signed Sqrt : Sqrt  SaturateOnIntegerOverflow=on
  RMS_Signal : Outport
  wires:
  Signed Sqrt/1 -> RMS_Signal/1
  Discrete  Mean value6/1 -> Signed Sqrt/1
  Product3/1 -> Discrete  Mean value6/1
  Signal/1 -> Product3/2, Product3/1

== system BANSHEE_SYSTEM/SC_ctrl/Overall/currents/RMS_Calculator2 ==
  Signal : Inport
  Discrete  Mean value6 : powerlib_extras/Discrete Measurements/Discrete  Mean value  Freq=60  Vinit=0  Ts=Ts
  Product3 : Product  RndMeth=Zero
  Signed Sqrt : Sqrt  SaturateOnIntegerOverflow=on
  RMS_Signal : Outport
  wires:
  Signed Sqrt/1 -> RMS_Signal/1
  Discrete  Mean value6/1 -> Signed Sqrt/1
  Product3/1 -> Discrete  Mean value6/1
  Signal/1 -> Product3/2, Product3/1
